simulink model "Enceinte_climatique_avec_correcteur_R2024b"  (R2024b)
settings: Solver=VariableStepAuto  StartTime=0.0  StopTime=10.0  RelTol=1e-3
undefined symbols (not defined in the file): dspblkCoreblockFVToolHelper, gcbh
settings Model: Creator=rofte  LastModifiedBy=elio
settings ConfigComp: CovBoundaryAbsTol=1.0e-5

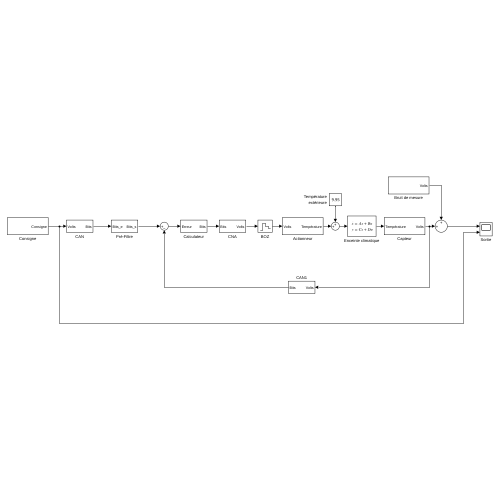
[thumbnail: Simulink's stored preview of the top-level diagram]
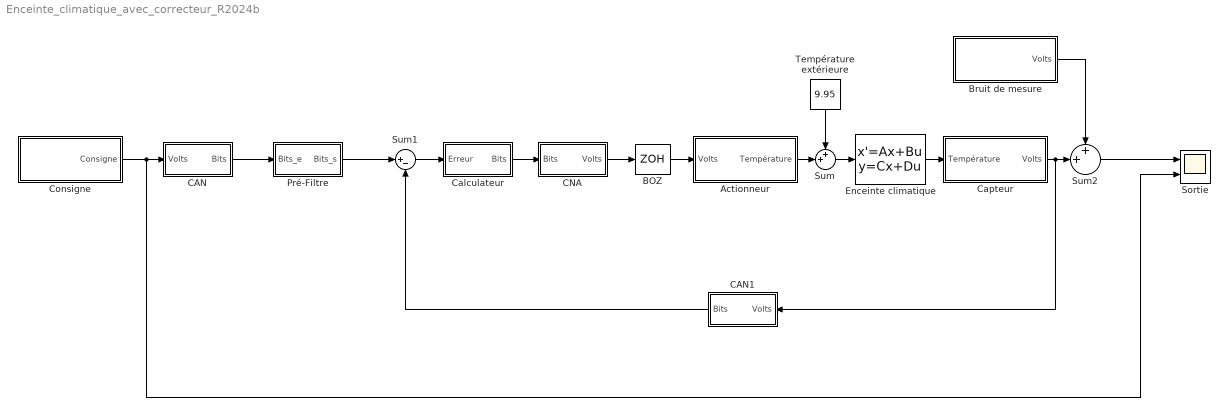
== system Enceinte_climatique_avec_correcteur_R2024b ==
  Actionneur : Subsystem
  BOZ : ZeroOrderHold  SampleTime=0.01
  Bruit de mesure : Subsystem
  CAN : Subsystem
  CAN1 : Subsystem
  CNA : Subsystem
  Calculateur : Subsystem
  Capteur : Subsystem
  Consigne : Subsystem
  Enceinte climatique : StateSpace  A=-2  B=2  D=0  InitialCondition=9.95
  Pré-Filtre : Subsystem
  Sortie : Scope  NumInputPorts=2
  Sum : Sum  Inputs=++|
  Sum1 : Sum  Inputs=|+-
  Sum2 : Sum  Inputs=++|
  Température extérieure : Constant  Value=9.95
  wires:
  Enceinte climatique/1 -> Capteur/1(Température)
  Capteur/1(Volts) -> CAN1/1(Volts), Sum2/2
  Actionneur/1(Température) -> Sum/2
  Sum/1 -> Enceinte climatique/1
  Sum2/1 -> Sortie/1
  Température extérieure/1 -> Sum/1
  CNA/1(Volts) -> BOZ/1
  BOZ/1 -> Actionneur/1(Volts)
  Calculateur/1(Bits) -> CNA/1(Bits)
  Consigne/1(Consigne) -> CAN/1(Volts), Sortie/2
  CAN1/1(Bits) -> Sum1/2
  Sum1/1 -> Calculateur/1(Erreur)
  CAN/1(Bits) -> Pré-Filtre/1(Bits_e)
  Pré-Filtre/1(Bits_s) -> Sum1/1
  Bruit de mesure/1(Volts) -> Sum2/1

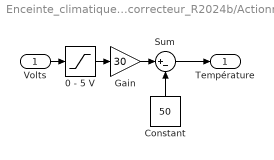
== system Enceinte_climatique_avec_correcteur_R2024b/Actionneur ==
  Volts : Inport
  "0 - 5 V " : Saturate  UpperLimit=5  LowerLimit=0
  Constant : Constant  Value=50
  Gain : Gain  Gain=30
  Sum : Sum  Inputs=|+-
  Température : Outport
  wires:
  Volts/1 -> "0 - 5 V "/1
  "0 - 5 V "/1 -> Gain/1
  Gain/1 -> Sum/1
  Constant/1 -> Sum/2
  Sum/1 -> Température/1

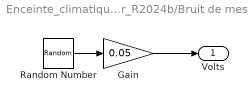
== system Enceinte_climatique_avec_correcteur_R2024b/Bruit de mesure ==
  Gain : Gain  Gain=0.05
  Random Number : RandomNumber  Variance=0.5  SampleTime=0.01
  Volts : Outport
  wires:
  Random Number/1 -> Gain/1
  Gain/1 -> Volts/1

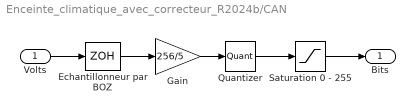
== system Enceinte_climatique_avec_correcteur_R2024b/CAN ==
  Volts : Inport
  Echantillonneur par BOZ : ZeroOrderHold  SampleTime=0.01
  Gain : Gain  Gain=256/5  SaturateOnIntegerOverflow=on  OutDataTypeStr=Inherit: Same as input  ParamDataTypeStr=Inherit: Same as input
  Quantizer : Quantizer  QuantizationInterval=1
  Saturation 0 - 255 : Saturate  UpperLimit=255  LowerLimit=0
  Bits : Outport
  wires:
  Volts/1 -> Echantillonneur par BOZ/1
  Gain/1 -> Quantizer/1
  Echantillonneur par BOZ/1 -> Gain/1
  Quantizer/1 -> Saturation 0 - 255/1
  Saturation 0 - 255/1 -> Bits/1

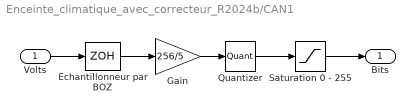
== system Enceinte_climatique_avec_correcteur_R2024b/CAN1 ==
  Volts : Inport
  Echantillonneur par BOZ : ZeroOrderHold  SampleTime=0.01
  Gain : Gain  Gain=256/5  SaturateOnIntegerOverflow=on  OutDataTypeStr=Inherit: Same as input  ParamDataTypeStr=Inherit: Same as input
  Quantizer : Quantizer  QuantizationInterval=1
  Saturation 0 - 255 : Saturate  UpperLimit=255  LowerLimit=0
  Bits : Outport
  wires:
  Volts/1 -> Echantillonneur par BOZ/1
  Gain/1 -> Quantizer/1
  Echantillonneur par BOZ/1 -> Gain/1
  Quantizer/1 -> Saturation 0 - 255/1
  Saturation 0 - 255/1 -> Bits/1

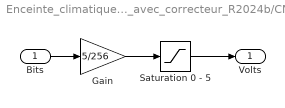
== system Enceinte_climatique_avec_correcteur_R2024b/CNA ==
  Bits : Inport
  Gain : Gain  Gain=5/256  SaturateOnIntegerOverflow=on  OutDataTypeStr=Inherit: Same as input  ParamDataTypeStr=Inherit: Same as input
  Saturation 0 - 5 : Saturate  UpperLimit=5  LowerLimit=0
  Volts : Outport
  wires:
  Bits/1 -> Gain/1
  Gain/1 -> Saturation 0 - 5/1
  Saturation 0 - 5/1 -> Volts/1

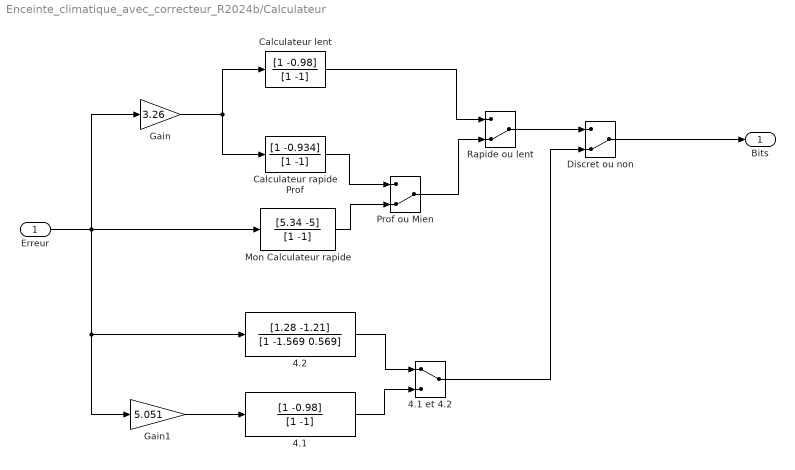
== system Enceinte_climatique_avec_correcteur_R2024b/Calculateur ==
  Erreur : Inport
  4.1 : DiscreteFilter  LoadFcn=dspblkCoreblockFVToolHelper(gcbh,'load');  Numerator=[1 -0.98]  Denominator=[1 -1]  SampleTime=0.01
      settings: CopyFcn=dspblkCoreblockFVToolHelper(gcbh,'copy');  DeleteFcn=dspblkCoreblockFVToolHelper(gcbh,'close');  ModelCloseFcn=dspblkCoreblockFVToolHelper(gcbh,'close');  PreSaveFcn=dspblkCoreblockFVToolHelper(gcbh,'presave');  PostSaveFcn=dspblkCoreblockFVToolHelper(gcbh,'postsave');  CloseFcn=dspblkCoreblockFVToolHelper(gcbh,'close');
  4.1 et 4.2 : ManualSwitch
  4.2 : DiscreteFilter  LoadFcn=dspblkCoreblockFVToolHelper(gcbh,'load');  Numerator=[1.28 -1.21]  Denominator=[1 -1.569 0.569]  SampleTime=0.01
      settings: CopyFcn=dspblkCoreblockFVToolHelper(gcbh,'copy');  DeleteFcn=dspblkCoreblockFVToolHelper(gcbh,'close');  ModelCloseFcn=dspblkCoreblockFVToolHelper(gcbh,'close');  PreSaveFcn=dspblkCoreblockFVToolHelper(gcbh,'presave');  PostSaveFcn=dspblkCoreblockFVToolHelper(gcbh,'postsave');  CloseFcn=dspblkCoreblockFVToolHelper(gcbh,'close');
  Calculateur lent : DiscreteFilter  LoadFcn=dspblkCoreblockFVToolHelper(gcbh,'load');  Numerator=[1 -0.98]  Denominator=[1 -1]  SampleTime=0.01
      settings: CopyFcn=dspblkCoreblockFVToolHelper(gcbh,'copy');  DeleteFcn=dspblkCoreblockFVToolHelper(gcbh,'close');  ModelCloseFcn=dspblkCoreblockFVToolHelper(gcbh,'close');  PreSaveFcn=dspblkCoreblockFVToolHelper(gcbh,'presave');  PostSaveFcn=dspblkCoreblockFVToolHelper(gcbh,'postsave');  CloseFcn=dspblkCoreblockFVToolHelper(gcbh,'close');
  Calculateur rapide Prof : DiscreteFilter  LoadFcn=dspblkCoreblockFVToolHelper(gcbh,'load');  Numerator=[1 -0.934]  Denominator=[1 -1]  SampleTime=0.01
      settings: CopyFcn=dspblkCoreblockFVToolHelper(gcbh,'copy');  DeleteFcn=dspblkCoreblockFVToolHelper(gcbh,'close');  ModelCloseFcn=dspblkCoreblockFVToolHelper(gcbh,'close');  PreSaveFcn=dspblkCoreblockFVToolHelper(gcbh,'presave');  PostSaveFcn=dspblkCoreblockFVToolHelper(gcbh,'postsave');  CloseFcn=dspblkCoreblockFVToolHelper(gcbh,'close');
  Discret ou non : ManualSwitch  CurrentSetting=0
  Gain : Gain  Gain=3.26
  Gain1 : Gain  Gain=5.051
  Mon Calculateur rapide : DiscreteFilter  LoadFcn=dspblkCoreblockFVToolHelper(gcbh,'load');  Numerator=[5.34 -5]  Denominator=[1 -1]  SampleTime=0.01
      settings: CopyFcn=dspblkCoreblockFVToolHelper(gcbh,'copy');  DeleteFcn=dspblkCoreblockFVToolHelper(gcbh,'close');  ModelCloseFcn=dspblkCoreblockFVToolHelper(gcbh,'close');  PreSaveFcn=dspblkCoreblockFVToolHelper(gcbh,'presave');  PostSaveFcn=dspblkCoreblockFVToolHelper(gcbh,'postsave');  CloseFcn=dspblkCoreblockFVToolHelper(gcbh,'close');
  Prof ou Mien : ManualSwitch  CurrentSetting=0
  Rapide ou lent : ManualSwitch  CurrentSetting=0
  Bits : Outport
  wires:
  Erreur/1 -> Gain/1, Mon Calculateur rapide/1, Gain1/1, 4.2/1
  Calculateur lent/1 -> Rapide ou lent/1
  Gain/1 -> Calculateur rapide Prof/1, Calculateur lent/1
  Mon Calculateur rapide/1 -> Prof ou Mien/2
  Calculateur rapide Prof/1 -> Prof ou Mien/1
  Prof ou Mien/1 -> Rapide ou lent/2
  Rapide ou lent/1 -> Discret ou non/1
  Discret ou non/1 -> Bits/1
  Gain1/1 -> 4.1/1
  4.1/1 -> 4.1 et 4.2/2
  4.2/1 -> 4.1 et 4.2/1
  4.1 et 4.2/1 -> Discret ou non/2

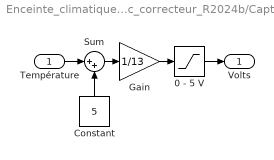
== system Enceinte_climatique_avec_correcteur_R2024b/Capteur ==
  Température : Inport
  "0 - 5 V " : Saturate  UpperLimit=5  LowerLimit=0
  Constant : Constant  Value=5
  Gain : Gain  Gain=1/13
  Sum : Sum  Inputs=|++
  Volts : Outport
  wires:
  Constant/1 -> Sum/2
  Température/1 -> Sum/1
  Sum/1 -> Gain/1
  Gain/1 -> "0 - 5 V "/1
  "0 - 5 V "/1 -> Volts/1

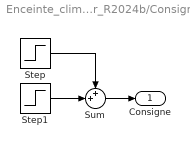
== system Enceinte_climatique_avec_correcteur_R2024b/Consigne ==
  Step : Step  Time=4  After=-0.5  SampleTime=0
  Step1 : Step  Time=0.5  Before=1.66  After=2.33  SampleTime=0
  Sum : Sum  Inputs=++|
  Consigne : Outport
  wires:
  Step/1 -> Sum/1
  Step1/1 -> Sum/2
  Sum/1 -> Consigne/1

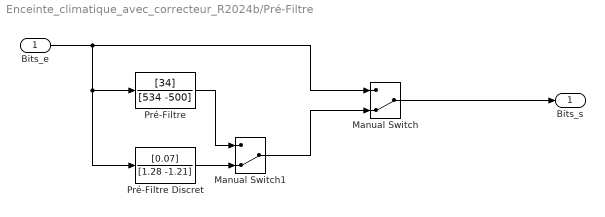
== system Enceinte_climatique_avec_correcteur_R2024b/Pré-Filtre ==
  Bits_e : Inport
  Manual Switch : ManualSwitch  CurrentSetting=0
  Manual Switch1 : ManualSwitch  CurrentSetting=0
  Pré-Filtre : DiscreteFilter  LoadFcn=dspblkCoreblockFVToolHelper(gcbh,'load');  Numerator=[34]  Denominator=[534 -500]  SampleTime=0.01
      settings: CopyFcn=dspblkCoreblockFVToolHelper(gcbh,'copy');  DeleteFcn=dspblkCoreblockFVToolHelper(gcbh,'close');  ModelCloseFcn=dspblkCoreblockFVToolHelper(gcbh,'close');  PreSaveFcn=dspblkCoreblockFVToolHelper(gcbh,'presave');  PostSaveFcn=dspblkCoreblockFVToolHelper(gcbh,'postsave');  CloseFcn=dspblkCoreblockFVToolHelper(gcbh,'close');
  Pré-Filtre Discret : DiscreteFilter  LoadFcn=dspblkCoreblockFVToolHelper(gcbh,'load');  Numerator=[0.07]  Denominator=[1.28 -1.21]  SampleTime=0.01
      settings: CopyFcn=dspblkCoreblockFVToolHelper(gcbh,'copy');  DeleteFcn=dspblkCoreblockFVToolHelper(gcbh,'close');  ModelCloseFcn=dspblkCoreblockFVToolHelper(gcbh,'close');  PreSaveFcn=dspblkCoreblockFVToolHelper(gcbh,'presave');  PostSaveFcn=dspblkCoreblockFVToolHelper(gcbh,'postsave');  CloseFcn=dspblkCoreblockFVToolHelper(gcbh,'close');
  Bits_s : Outport
  wires:
  Bits_e/1 -> Pré-Filtre/1, Pré-Filtre Discret/1, Manual Switch/1
  Manual Switch/1 -> Bits_s/1
  Pré-Filtre/1 -> Manual Switch1/1
  Manual Switch1/1 -> Manual Switch/2
  Pré-Filtre Discret/1 -> Manual Switch1/2
